simulink model "CAMFC2_Quad_New_02"  (R2017b)
settings: Solver=ode45  StartTime=0.0  StopTime=600  RelTol=1e-3  EnableMultiTasking=on
InitFcn:
  | constant_CAMFC2_Quad_New_02
values from neighbouring files (symbols this model uses):
  alpha = 0.1    [constant_CAMFC2_01_WMR01.m]    (also in constant_CAMFC2_04_Comp.m = 0.01; constant_CAMFC2_04_Quad_03.m; constant_CAMFC2_04_Simple.m = 0.01; constant_CAMFC2_04_Simple_DoubleIntegrator.m = 0.01)
  AN = [     0 1 0 0 ... (first row only)    [constant_CAMFC2_01_WMR01.m]    (also in constant_CAMFC2_04_Comp.m = [     0 1 0 0 1; constant_CAMFC2_04_Quad_03.m; constant_CAMFC2_04_Simple.m; constant_CAMFC2_04_Simple_DoubleIntegrator.m)
  B = eye(n)    [constant_CAMFC2_01_WMR01.m]    (also in constant_CAMFC2_04_Quad_03.m; constant_CAMFC2_Quad_New_02.m)
  B_pseudo_inverse = ((B'*B)^(-1))*B'    [constant_CAMFC2_01_WMR01.m]    (also in constant_CAMFC2_Quad_New_02.m)
  BBT_inv = ((B'*B)^(-1))*B'    [constant_CAMFC2_04_Quad_03.m]    (also in constant_CAMFC2_Quad_New_02.m)
  Beta = 0.2    [constant_CAMFC2_04_Quad_03.m]    (also in constant_CAMFC2_Quad_New_02.m = 0.1)
  BN = [     1 0 0 0 ... (first row only)    [constant_CAMFC2_01_WMR01.m]    (also in constant_CAMFC2_04_Comp.m = [     0 0 0 0 0; constant_CAMFC2_04_Quad_03.m; constant_CAMFC2_04_Simple.m; constant_CAMFC2_04_Simple_DoubleIntegrator.m)
  epsilon_struct = struct('data',epsilon_InitVal)    [constant_CAMFC2_01_WMR01.m]    (also in constant_CAMFC2_04_Comp.m; constant_CAMFC2_04_Quad_03.m; constant_CAMFC2_04_Simple.m; constant_CAMFC2_04_Simple_DoubleIntegrator.m)
  gama1 = 1e4*diag([1e-6*ones(2,1);1e0*ones(2,1)])    [constant_CAMFC2_01_WMR01.m]    (also in constant_CAMFC2_04_Comp.m = 1e+3*diag([1e-6;1e-0]); constant_CAMFC2_04_Quad_03.m = 1e+2*diag(1e-0*ones(n0,1)); constant_CAMFC2_04_Simple.m = 1e+2*diag([1e-0;1e-0]); constant_CAMFC2_04_Simple_Formation.m = 1e+2*diag([1e-0;1e-0]))
  gama2 = 1e-2*diag([1e-6*ones(2,1);1e0*ones(2,1)])    [constant_CAMFC2_01_WMR01.m]    (also in constant_CAMFC2_04_Comp.m = 1e+0*diag([1e-6;1e-0]); constant_CAMFC2_04_Quad_03.m = 1e+0*diag(1e-0*ones(n0,1)); constant_CAMFC2_04_Simple.m = 1e+1*diag([1e-0;1e-0]); constant_CAMFC2_04_Simple_Formation.m = 1e+1*diag([1e-0;1e-0]))
  gamma_0 = 1e+0*diag([1e-0*ones(n0,1);1e-0*ones(n0,1)])    [constant_CAMFC2_04_Quad_03.m]    (also in constant_CAMFC2_Quad_New_02.m = 1e-2*diag([1e-6*ones(n0,1);1e-0*ones(n0,1)]))
  gamma_1 = 1e+2*diag([1e-0*ones(n0,1);1e-0*ones(n0,1)])    [constant_CAMFC2_04_Quad_03.m]    (also in constant_CAMFC2_Quad_New_02.m = 1e+1*diag([1e-6*ones(n0,1);1e-0*ones(n0,1)]))
  ge = 9.81    [constant_CAMFC2_04_Comp.m]    (also in constant_CAMFC2_04_Quad_03.m; constant_CAMFC2_04_Simple.m; constant_CAMFC2_04_Simple_DoubleIntegrator.m; constant_CAMFC2_04_Simple_DoubleIntegrator_02.m)
  H = L + BN    [constant_CAMFC2_01_WMR01.m]    (also in constant_CAMFC2_04_Comp.m; constant_CAMFC2_04_Quad_03.m; constant_CAMFC2_04_Simple.m; constant_CAMFC2_04_Simple_DoubleIntegrator.m)
  J = 0.01    [constant_CAMFC2_01_WMR01.m]    (also in constant_CAMFC2_04_Quad_03.m = 1.0e-3 * diag([1 1 2],0); constant_CAMFC2_Quad_New_02.m = 1.2416e-3 * diag([1 1 2],0))
  K = 1e-2*eye(n)    [constant_CAMFC2_01_WMR01.m]    (also in constant_CAMFC2_Quad_New_02.m = 1e+1*eye(n))
  k1 = 1    [constant_CAMFC2_01_WMR01.m]    (also in constant_CAMFC2_04_Comp.m; constant_CAMFC2_04_Quad_03.m = 50; constant_CAMFC2_04_Simple.m; constant_CAMFC2_04_Simple_DoubleIntegrator.m)
  k2 = 1    [constant_CAMFC2_01_WMR01.m]    (also in constant_CAMFC2_04_Comp.m; constant_CAMFC2_04_Quad_03.m; constant_CAMFC2_04_Simple.m; constant_CAMFC2_04_Simple_DoubleIntegrator.m)
  Ka = 0.1    [constant_CAMFC2_04_Quad_03.m]    (also in constant_CAMFC2_Quad_New_02.m = 0.01)
  Kd = 0.1    [constant_CAMFC2_04_Quad_03.m]    (also in constant_CAMFC2_Quad_New_02.m = 0.01)
  Kf = 1e-5    (= 1e-05)    [constant_CAMFC2_Quad_New_02.m]
  Kt = 0.01 * Kf    (= 1e-07)    [constant_CAMFC2_Quad_New_02.m]
  Lq = 1    [constant_CAMFC2_04_Quad_03.m]    (also in constant_CAMFC2_Quad_New_02.m = 0.2)
  m = 6    [constant_CAMFC2_04_Quad_03.m]    (also in constant_CAMFC2_Quad_New_02.m)
  M = 1    [constant_CAMFC2_01_WMR01.m]    (also in constant_CAMFC2_04_Quad_03.m = 2; constant_CAMFC2_Quad_New_02.m = 2)
  N = 4    [constant_CAMFC2_01_WMR01.m]    (also in constant_CAMFC2_04_Comp.m = 5; constant_CAMFC2_04_Quad_03.m; constant_CAMFC2_04_Simple.m; constant_CAMFC2_04_Simple_DoubleIntegrator.m)
  n = 4    [constant_CAMFC2_01_WMR01.m]    (also in constant_CAMFC2_04_Comp.m = 2; constant_CAMFC2_04_Quad_03.m = 6; constant_CAMFC2_04_Simple.m = 2; constant_CAMFC2_04_Simple_DoubleIntegrator.m = 2)
  n0 = 2    [constant_CAMFC2_01_WMR01.m]    (also in constant_CAMFC2_04_Comp.m = 1; constant_CAMFC2_04_Quad_03.m = 3; constant_CAMFC2_04_Simple.m; constant_CAMFC2_04_Simple_DoubleIntegrator.m = 1)
  Observer_Gain = 100    [constant_CAMFC2_01_WMR01.m]    (also in constant_CAMFC2_04_Comp.m = 10; constant_CAMFC2_04_Quad_03.m = 1; constant_CAMFC2_04_Simple.m; constant_CAMFC2_04_Simple_DoubleIntegrator.m)
  Observer_Gain1 = 100    [constant_CAMFC2_01_WMR01.m]    (also in constant_CAMFC2_04_Comp.m = 10; constant_CAMFC2_04_Quad_03.m = 1; constant_CAMFC2_04_Simple.m; constant_CAMFC2_04_Simple_DoubleIntegrator.m)
  P_struct = struct('data',P_InitVal)    [constant_CAMFC2_01_WMR01.m]    (also in constant_CAMFC2_04_Comp.m; constant_CAMFC2_04_Quad_03.m; constant_CAMFC2_04_Simple.m; constant_CAMFC2_04_Simple_DoubleIntegrator.m)
  Q = 1e-0*eye(n)    [constant_CAMFC2_01_WMR01.m]    (also in constant_CAMFC2_04_Comp.m = 1.0e+2*eye(n); constant_CAMFC2_04_Quad_03.m = 1e-0*eye(n0); constant_CAMFC2_04_Simple.m = 1.0e+1*eye(n); constant_CAMFC2_04_Simple_Formation.m = 1.0e+1*eye(n))
  QR = 1e-0*eye(n)    [constant_CAMFC2_04_Quad_03.m]    (also in constant_CAMFC2_Quad_New_02.m = 1e+0*eye(n))
  R = 1e-0*eye(n)    [constant_CAMFC2_01_WMR01.m]    (also in constant_CAMFC2_04_Quad_03.m; constant_CAMFC2_Quad_New_02.m = 1e+0*eye(n))
  r_formX = 1.0    (= 1)    [constant_CAMFC2_04_Quad_03.m]    (also in constant_CAMFC2_Quad_New_02.m)
  r_formY = 1.0    (= 1)    [constant_CAMFC2_04_Quad_03.m]    (also in constant_CAMFC2_Quad_New_02.m)
  r_formZ = 0.5    [constant_CAMFC2_04_Quad_03.m]    (also in constant_CAMFC2_Quad_New_02.m = 1)
  rho1 = 1e-1    (= 0.1)    [constant_CAMFC2_01_WMR01.m]    (also in constant_CAMFC2_04_Comp.m = 1; constant_CAMFC2_04_Quad_03.m = 1; constant_CAMFC2_04_Simple.m = 1; constant_CAMFC2_04_Simple_DoubleIntegrator.m = 1)
  rho2 = 1e-3    (= 0.001)    [constant_CAMFC2_01_WMR01.m]    (also in constant_CAMFC2_04_Comp.m = 1; constant_CAMFC2_04_Quad_03.m = 1; constant_CAMFC2_04_Simple.m = 1; constant_CAMFC2_04_Simple_DoubleIntegrator.m = 10)
  rho_0 = 1e-0    (= 1)    [constant_CAMFC2_04_Quad_03.m]    (also in constant_CAMFC2_Quad_New_02.m = 0.01)
  rho_1 = 1e-0    (= 1)    [constant_CAMFC2_04_Quad_03.m]    (also in constant_CAMFC2_Quad_New_02.m = 0.01)
  T_struct = struct('data',T_InitVal)    [constant_CAMFC2_01_WMR01.m]    (also in constant_CAMFC2_04_Comp.m; constant_CAMFC2_04_Quad_03.m; constant_CAMFC2_04_Simple.m; constant_CAMFC2_04_Simple_DoubleIntegrator.m)
  U_dot0_M = U_dot0_m*ones(n,1)    [constant_CAMFC2_01_WMR01.m]    (also in constant_CAMFC2_Quad_New_02.m = U_dot0_m*ones(n0,1))
  Upsilon_M = Upsilon_m*ones(n,1)    [constant_CAMFC2_01_WMR01.m]    (also in constant_CAMFC2_04_Comp.m; constant_CAMFC2_04_Quad_03.m = Upsilon_m*ones(n0,1); constant_CAMFC2_04_Simple.m; constant_CAMFC2_04_Simple_DoubleIntegrator.m)
  X_M = X_m*ones(n0,1)    [constant_CAMFC2_Quad_New_02.m]
(part 3 of 3)

== matlab function CAMFC2_Quad_New_02/Agent #4/Decenteralized Cooperaive Controller #4/Cooperative Observers #1/Differentiator2/Sliding differentiator1 ==
  data: Du1 output; e input; k2 parameter; alpha parameter
function Du1 = fcn(e,k2,alpha)

a=k2;

ABS = abs(e);
SGN = e ./ (ABS + alpha);
Du1 = - a*SGN;

end

== matlab function CAMFC2_Quad_New_02/Agent #4/Decenteralized Cooperaive Controller #4/Cooperative Observers #1/Observer T#4 ==
  data: T_struct parameter; T input; DT_i output; epsilon input; epsilon_struct parameter; H parameter; BN parameter; AN parameter; T_i input; Upsilon_M parameter; epsilon_i output; N parameter; n0 parameter; Agent_Num input; Observer_Gain1 parameter; chi input
function [DT_i,epsilon_i] = fcn(T_struct,T,epsilon,epsilon_struct,H,BN,AN,T_i,Upsilon_M,N,n0,Agent_Num,Observer_Gain1, chi)

T_struct(1).data = T.t1;
T_struct(2).data = T.t2;
T_struct(3).data = T.t3;
T_struct(4).data = T.t4;

epsilon_struct(1).data = epsilon.eps1;
epsilon_struct(2).data = epsilon.eps2;
epsilon_struct(3).data = epsilon.eps3;
epsilon_struct(4).data = epsilon.eps4;

epsilon_i = + BN(Agent_Num,Agent_Num)*(T_i - chi);
Sum2 = zeros(N+1,n0);
for i=1:N
    epsilon_i = epsilon_i + ( AN(Agent_Num,i) * (T_i - T_struct(i).data) );  
    Sum2 = Sum2 + ( H(i,Agent_Num) * epsilon_struct(i).data );
end

Sum21 = abs(Sum2) + 0.1;
SGN2 = Sum2./Sum21;

DT_i = -Observer_Gain1*epsilon_i - SGN2*diag(Upsilon_M);

end

== matlab function CAMFC2_Quad_New_02/Agent #4/Decenteralized Cooperaive Controller #4/Cooperative Observers #1/Observer q#4 ==
  data: q input; Dq_i output; tau input; H parameter; BN parameter; AN parameter; q_i input; u0 input; U_dot0_M parameter; tau_i output; N parameter; Agent_Num input; Observer_Gain parameter; n0 parameter; alpha parameter
function [Dq_i,tau_i] = fcn(q,tau,H,BN,AN,q_i,u0,U_dot0_M,N,Agent_Num,Observer_Gain,n0,alpha)

tau_i = + BN(Agent_Num,Agent_Num)*(q_i - u0);
Sum2 = zeros(n0,1);
for i=1:N
    tau_i = tau_i + ( AN(Agent_Num,i) * (q_i - q(((i-1)*n0+1):n0*i)) );  
    Sum2 = Sum2 + ( H(i,Agent_Num) * tau(((i-1)*n0+1):n0*i) );
end

Sum21 = abs(Sum2) + alpha;
SGN2 = Sum2./Sum21;

Dq_i = -Observer_Gain*tau_i - diag(SGN2)*U_dot0_M;

end

== matlab function CAMFC2_Quad_New_02/Agent #4/Decenteralized Cooperaive Controller #4/Cooperative Observers #1/Observer x0_hat#4 ==
  data: x0_hat input; Dx0_hat_i output; x0_tilde input; H parameter; BN parameter; AN parameter; x0_hat_i input; x0 input; X_M parameter; x0_tilde_i output; N parameter; Agent_Num input; Observer_Gain parameter; n0 parameter; alpha parameter
function [Dx0_hat_i,x0_tilde_i] = fcn(x0_hat,x0_tilde,H,BN,AN,x0_hat_i,x0,X_M,N,Agent_Num,Observer_Gain,n0,alpha)

x0_tilde_i = + BN(Agent_Num,Agent_Num)*(x0_hat_i - x0);
Sum2 = zeros(n0,1);
for i=1:N
    x0_tilde_i = x0_tilde_i + ( AN(Agent_Num,i) * (x0_hat_i - x0_hat(((i-1)*n0+1):n0*i)) );  
    Sum2 = Sum2 + ( H(i,Agent_Num) * x0_tilde(((i-1)*n0+1):n0*i) );
end

Sum21 = abs(Sum2) + alpha;
SGN2 = Sum2./Sum21;

Dx0_hat_i = -Observer_Gain*x0_tilde_i - diag(SGN2)*X_M;

end

== matlab function CAMFC2_Quad_New_02/Agent #4/Decenteralized Cooperaive Controller #4/Rotational/Differentiator/Sliding differentiator1 ==
  data: Du1 output; e input; n parameter; k2 parameter
function Du1 = fcn(e,n,k2)

a=k2;

ABS = zeros(n,1);
for i=1:n
    if e(i)>0
        ABS(i) = e(i);
    else
        ABS(i) = -e(i);
    end
end
SGN = e ./ (ABS + 0.01);

Du1 = - a*SGN;

end

== matlab function CAMFC2_Quad_New_02/Agent #4/Decenteralized Cooperaive Controller #4/Rotational/g-Estimator ==
  data: sigma input; g_hat input; P input; rho_1 parameter; gamma_1 parameter; Dg_hat output
function Dg_hat = fcn(sigma,g_hat,P,rho_1,gamma_1)

Dg_hat = - gamma_1 * P * sigma - rho_1 * gamma_1 * g_hat;

end

== matlab function CAMFC2_Quad_New_02/Agent #4/Decenteralized Cooperaive Controller #4/Rotational/g-Estimator1 ==
  data: sigma input; x input; P input; rho_0 parameter; gamma_0 parameter; Da_hat output; a_hat input
function Da_hat = fcn(sigma,x,P,rho_0,gamma_0,a_hat)

DVa_hat = - gamma_0 * P * diag(sigma) * (x - sigma) - rho_0 * gamma_0 * diag(a_hat);

Da_hat = diag(DVa_hat);

end

== matlab function CAMFC2_Quad_New_02/Agent #4/Decenteralized Cooperaive Controller #4/Rotational/main ==
  data: sigma input; zeta input; u output; Dy_d input; R parameter; P input; a_hat input; B parameter; g_hat input; x input; QR parameter; BBT_inv parameter; n parameter
function u = fcn(sigma,zeta,Dy_d,R,P,a_hat,B,g_hat,x,QR,BBT_inv,n)

u1 = (1/2) * R * B' * P * sigma;
u2 = BBT_inv * (Dy_d - a_hat*x + (eye(n) + 2*(((P)^(-1)*QR)) + a_hat)*sigma - g_hat - zeta) - (3/4) * R * B' * P * sigma;

u = u1 + u2;

end

== matlab function CAMFC2_Quad_New_02/Agent #4/Decenteralized Cooperaive Controller #4/Rotational/variable change ==
  data: X input; Xd input; x_mod output; u input; xd_mod output; e_mod output
function [x_mod,xd_mod,e_mod] = fcn(X,Xd,u)

x_mod = [X(4:6);X(10:12)];

xd_mod = [Xd;u(1:3)];

e_mod = xd_mod - x_mod;


end

== matlab function CAMFC2_Quad_New_02/Agent #1/Decenteralized Cooperaive Controller #1/Rotational/CARE ==
  data: P input; a_hat input; B parameter; R parameter; DP output; QR parameter
function DP = fcn(P,a_hat,B,R,QR)

DP = a_hat*P + P*a_hat' - P*B*R*B'*P + 2*QR;

end

== matlab function CAMFC2_Quad_New_02/Data Bus /Reference Trajectory/Differentiator0/Sliding differentiator ==
  data: u output; u1 input; e input; k1 parameter; alpha parameter
function u = fcn(u1,e,k1,alpha)

b=k1;

ABS = abs(e);
SGN = e ./ (ABS + alpha);
u = u1 - b*((ABS.^0.5).*SGN); 

end

== matlab function CAMFC2_Quad_New_02/Data Bus /Translational Log/For matrix Plot1/MATLAB Function ==
  data: u input; y output
function y = fcn(u)
S1 = size(u,1);
S2 = size(u,2);

y = zeros(S1*S2,1);
num = 0;
for i=1:S1
    for j=1:S2
        num = num + 1;
        y(num,1) = u(i,j);
    end
end

end

== matlab function CAMFC2_Quad_New_02/Data Bus /Translational Log/For matrix Plot2/MATLAB Function ==
  data: u input; y output
function y = fcn(u)
S1 = size(u,1);
S2 = size(u,2);

y = zeros(S1*S2,1);
num = 0;
for i=1:S1
    for j=1:S2
        num = num + 1;
        y(num,1) = u(i,j);
    end
end

end

== matlab function CAMFC2_Quad_New_02/Data Bus /Translational Log/For matrix Plot3/MATLAB Function ==
  data: u input; y output
function y = fcn(u)
S1 = size(u,1);
S2 = size(u,2);

y = zeros(S1*S2,1);
num = 0;
for i=1:S1
    for j=1:S2
        num = num + 1;
        y(num,1) = u(i,j);
    end
end

end

== matlab function CAMFC2_Quad_New_02/Data Bus /Translational Log/For matrix Plot4/MATLAB Function ==
  data: u input; y output
function y = fcn(u)
S1 = size(u,1);
S2 = size(u,2);

y = zeros(S1*S2,1);
num = 0;
for i=1:S1
    for j=1:S2
        num = num + 1;
        y(num,1) = u(i,j);
    end
end

end

== matlab function CAMFC2_Quad_New_02/Data Bus /Translational Log/For matrix Plot5/MATLAB Function ==
  data: u input; y output
function y = fcn(u)
S1 = size(u,1);
S2 = size(u,2);

y = zeros(S1*S2,1);
num = 0;
for i=1:S1
    for j=1:S2
        num = num + 1;
        y(num,1) = u(i,j);
    end
end

end

== matlab function CAMFC2_Quad_New_02/Data Bus /Translational Log/For matrix Plot6/MATLAB Function ==
  data: u input; y output
function y = fcn(u)
S1 = size(u,1);
S2 = size(u,2);

y = zeros(S1*S2,1);
num = 0;
for i=1:S1
    for j=1:S2
        num = num + 1;
        y(num,1) = u(i,j);
    end
end

end

== matlab function CAMFC2_Quad_New_02/Data Bus /Translational Log/For matrix Plot7/MATLAB Function ==
  data: u input; y output
function y = fcn(u)
S1 = size(u,1);
S2 = size(u,2);

y = zeros(S1*S2,1);
num = 0;
for i=1:S1
    for j=1:S2
        num = num + 1;
        y(num,1) = u(i,j);
    end
end

end

== matlab function CAMFC2_Quad_New_02/Data Bus /Observers Log/For matrix Plot8/MATLAB Function ==
  data: u input; y output
function y = fcn(u)
S1 = size(u,1);
S2 = size(u,2);

y = zeros(S1*S2,1);
num = 0;
for i=1:S1
    for j=1:S2
        num = num + 1;
        y(num,1) = u(i,j);
    end
end

end

== matlab function CAMFC2_Quad_New_02/Data Bus /Observers Log/For matrix Plot9/MATLAB Function ==
  data: u input; y output
function y = fcn(u)
S1 = size(u,1);
S2 = size(u,2);

y = zeros(S1*S2,1);
num = 0;
for i=1:S1
    for j=1:S2
        num = num + 1;
        y(num,1) = u(i,j);
    end
end

end

== matlab function CAMFC2_Quad_New_02/Agent #2/Decenteralized Cooperaive Controller #2/Rotational/CARE ==
  data: P input; a_hat input; B parameter; R parameter; DP output; QR parameter
function DP = fcn(P,a_hat,B,R,QR)

DP = a_hat*P + P*a_hat' - P*B*R*B'*P + 2*QR;

end

== matlab function CAMFC2_Quad_New_02/Agent #2/Decenteralized Cooperaive Controller #2/Rotational/Differentiator/Sliding differentiator ==
  data: u output; u1 input; e input; n parameter; k1 parameter
function u = fcn(u1,e,n,k1)

b=k1;

ABS = zeros(n,1);
for i=1:n
    if e(i)>0
        ABS(i) = e(i);
    else
        ABS(i) = -e(i);
    end
end
SGN = e ./ (ABS + 0.01);

u = u1 - b*(ABS.^0.5).*SGN;

end

== matlab function CAMFC2_Quad_New_02/Data Bus /Translational Log/For matrix Plot/MATLAB Function ==
  data: u input; y output
function y = fcn(u)
S1 = size(u,1);
S2 = size(u,2);

y = zeros(S1*S2,1);
num = 0;
for i=1:S1
    for j=1:S2
        num = num + 1;
        y(num,1) = u(i,j);
    end
end

end

== matlab function CAMFC2_Quad_New_02/Data Bus /Observers Log/For matrix Plot10/MATLAB Function ==
  data: u input; y output
function y = fcn(u)
S1 = size(u,1);
S2 = size(u,2);

y = zeros(S1*S2,1);
num = 0;
for i=1:S1
    for j=1:S2
        num = num + 1;
        y(num,1) = u(i,j);
    end
end

end

== matlab function CAMFC2_Quad_New_02/Data Bus /Observers Log/For matrix Plot11/MATLAB Function ==
  data: u input; y output
function y = fcn(u)
S1 = size(u,1);
S2 = size(u,2);

y = zeros(S1*S2,1);
num = 0;
for i=1:S1
    for j=1:S2
        num = num + 1;
        y(num,1) = u(i,j);
    end
end

end

== matlab function CAMFC2_Quad_New_02/Data Bus /Observers Log/For matrix Plot12/MATLAB Function ==
  data: u input; y output
function y = fcn(u)
S1 = size(u,1);
S2 = size(u,2);

y = zeros(S1*S2,1);
num = 0;
for i=1:S1
    for j=1:S2
        num = num + 1;
        y(num,1) = u(i,j);
    end
end

end

== matlab function CAMFC2_Quad_New_02/Agent #2/Decenteralized Cooperaive Controller #2/Rotational/Differentiator/Sliding differentiator1 ==
  data: Du1 output; e input; n parameter; k2 parameter
function Du1 = fcn(e,n,k2)

a=k2;

ABS = zeros(n,1);
for i=1:n
    if e(i)>0
        ABS(i) = e(i);
    else
        ABS(i) = -e(i);
    end
end
SGN = e ./ (ABS + 0.01);

Du1 = - a*SGN;

end

== matlab function CAMFC2_Quad_New_02/Data Bus /Observers Log/For matrix Plot13/MATLAB Function ==
  data: u input; y output
function y = fcn(u)
S1 = size(u,1);
S2 = size(u,2);

y = zeros(S1*S2,1);
num = 0;
for i=1:S1
    for j=1:S2
        num = num + 1;
        y(num,1) = u(i,j);
    end
end

end

== matlab function CAMFC2_Quad_New_02/Agent #2/Decenteralized Cooperaive Controller #2/Rotational/g-Estimator ==
  data: sigma input; g_hat input; P input; rho_1 parameter; gamma_1 parameter; Dg_hat output
function Dg_hat = fcn(sigma,g_hat,P,rho_1,gamma_1)

Dg_hat = - gamma_1 * P * sigma - rho_1 * gamma_1 * g_hat;

end

== matlab function CAMFC2_Quad_New_02/Agent #4/Plant #4/MATLAB Function ==
  data: X input; U input; t input; DX output; Kf parameter; Kt parameter; Kd parameter; Ka parameter; M parameter; J parameter; Lq parameter; ge parameter
function DX = fcn(X,U,t,Kf,Kt,Kd,Ka,M,J,Lq,ge)

phi = X(4);
theta = X(5);
psi = X(6);

Rq = [cos(psi)*cos(theta) -sin(psi)*cos(phi)+cos(psi)*sin(theta)*sin(phi) sin(psi)*sin(phi)+cos(psi)*sin(theta)*cos(phi);
    sin(psi)*cos(theta) cos(psi)*cos(phi)+sin(psi)*sin(theta)*sin(phi) -cos(psi)*sin(phi)+sin(psi)*sin(theta)*cos(phi);
    -sin(theta) cos(theta)*sin(phi) cos(theta)*cos(phi)]; 

R_omega = [1 0 -sin(theta);
    0 cos(phi) cos(theta)*sin(phi);
    0 -sin(phi) cos(theta)*cos(phi)];

EXT_PRD = External_Product3(X(10:12),(J*X(10:12)));

F1 = Kf * U(1)^2;
F2 = Kf * U(2)^2;
F3 = Kf * U(3)^2;
F4 = Kf * U(4)^2;
  
FT = F1 + F2 + F3 + F4;
 
T1 = Kt * U(1)^2;
T2 = Kt * U(2)^2;
T3 = Kt * U(3)^2;
T4 = Kt * U(4)^2;
 
TT1 = Lq*(F3-F1);
TT2 = Lq*(F4-F2);
TT3 = (T1-T2+T3-T4);

FTT = Rq * [0;0;FT];
FTx = FTT(1);
FTy = FTT(2);
FTz = FTT(3);

DP = X(7:9);
DPHI = (R_omega)^(-1) * X(10:12); 
Dv = (1/M)*([FTx;FTy;FTz] - Kd*X(7:9) - M*[0;0;ge]) + Rq*(0.1*sin(1*t))*[0;0;1]; 
Dw = (J^(-1))*([TT1;TT2;TT3] - Ka*X(10:12) - EXT_PRD) + (1*sin(1*t)*[1;1;1]);

DX = [DP;DPHI;Dv;Dw];

end

== matlab function CAMFC2_Quad_New_02/Data Bus /Observers Log/For matrix Plot14/MATLAB Function ==
  data: u input; y output
function y = fcn(u)
S1 = size(u,1);
S2 = size(u,2);

y = zeros(S1*S2,1);
num = 0;
for i=1:S1
    for j=1:S2
        num = num + 1;
        y(num,1) = u(i,j);
    end
end

end

== matlab function CAMFC2_Quad_New_02/Data Bus /Observers Log/For matrix Plot15/MATLAB Function ==
  data: u input; y output
function y = fcn(u)
S1 = size(u,1);
S2 = size(u,2);

y = zeros(S1*S2,1);
num = 0;
for i=1:S1
    for j=1:S2
        num = num + 1;
        y(num,1) = u(i,j);
    end
end

end

== matlab function CAMFC2_Quad_New_02/Data Bus /Reference Trajectory/Differentiator0/Sliding differentiator1 ==
  data: Du1 output; e input; k2 parameter; alpha parameter
function Du1 = fcn(e,k2,alpha)

a=k2;

ABS = abs(e);
SGN = e ./ (ABS + alpha);
Du1 = - a*SGN;

end

== matlab function CAMFC2_Quad_New_02/Data Bus /Reference Trajectory/MATLAB Function ==
  data: r_formZ_inp input; chi output; r_formX_inp input; r_formY_inp input
function chi = fcn(r_formZ_inp, r_formX_inp, r_formY_inp)

Delta_form = [...
    +r_formX_inp +r_formY_inp +r_formZ_inp;
    -r_formX_inp +r_formY_inp +2*r_formZ_inp;
    -r_formX_inp -r_formY_inp +3*r_formZ_inp;
    +r_formX_inp -r_formY_inp +4*r_formZ_inp];

chi = [0 0 0;
    Delta_form];

end

== matlab function CAMFC2_Quad_New_02/Agent #1/Decenteralized Cooperaive Controller #1/Rotational/Differentiator/Sliding differentiator ==
  data: u output; u1 input; e input; n parameter; k1 parameter
function u = fcn(u1,e,n,k1)

b=k1;

ABS = zeros(n,1);
for i=1:n
    if e(i)>0
        ABS(i) = e(i);
    else
        ABS(i) = -e(i);
    end
end
SGN = e ./ (ABS + 0.01);

u = u1 - b*(ABS.^0.5).*SGN;

end

== matlab function CAMFC2_Quad_New_02/Agent #4/Decenteralized Cooperaive Controller #4/Translational #4/Adaptive Law A_T #4 ==
  data: Agent_Num input; A_hat input; gama2 parameter; rho2 parameter; T_i input; P_i input; DA_hat output; e_i input; H parameter; BN parameter; N parameter; n parameter; n0 parameter; z0 input; x0_hat_inp input; ui input
function DA_hat = fcn(Agent_Num,A_hat,gama2,rho2,T_i,P_i,e_i,H,BN,N,n,n0,z0,x0_hat_inp,ui)

%% 
z0_i = [z0;ui(1:n0)]; 
x0_hat_i = [x0_hat_inp;ui(1:n0)];

%%
vA_hat = diag(A_hat);

Sum = zeros(n,1);
for i=2:(N+1)
    Sum = Sum + ( H(Agent_Num,(i-1)) * ( (2*x0_hat_i) - (2*[T_i(1,:)';zeros(n0,1)]) + ([T_i(i,:)';zeros(n0,1)]) ) );
end
Sum(1:n0) = Sum(1:n0) + ( BN(Agent_Num,Agent_Num)*z0_i(1:n0) ) - e_i(1:n0);
Sum(n0+1:n) = Sum(n0+1:n) + ( 1*z0_i(n0+1:n) ) - e_i(n0+1:n);
    
DvA_hat = -gama2*diag(Sum)*P_i * e_i - (rho2*gama2*vA_hat);

DA_hat = diag(DvA_hat);

end

== matlab function CAMFC2_Quad_New_02/Agent #4/Decenteralized Cooperaive Controller #4/Translational #4/Adaptive Law g_T #4 ==
  data: Agent_Num input; g_hat input; gama1 parameter; rho1 parameter; P input; P_struct parameter; Dg_hat output; e input; H parameter; N parameter; n parameter
function Dg_hat = fcn(Agent_Num,g_hat,gama1,rho1,P,P_struct,e,H,N,n)

P_struct(1).data = P.p1;
P_struct(2).data = P.p2;
P_struct(3).data = P.p3;
P_struct(4).data = P.p4;

Sum = zeros(n,1);
for i=1:N  
    Sum = Sum + (H(i,Agent_Num) * P_struct(i).data * e((i-1)*n+1:(i*n),1)); %Adaptive law
end
    
Dg_hat = -gama1*Sum - (rho1*gama1*g_hat);

end

== matlab function CAMFC2_Quad_New_02/Agent #4/Decenteralized Cooperaive Controller #4/Translational #4/DRE_T ==
  data: P input; A_hat input; B parameter; R parameter; DP output; Q parameter
function DP = fcn(P,A_hat,B,R,Q)

DP = 2*A_hat*P + 2*P*A_hat' - P*B*R*B'*P + 2*Q;

end

== matlab function CAMFC2_Quad_New_02/Agent #4/Decenteralized Cooperaive Controller #4/Translational #4/Differentiator1/Sliding differentiator ==
  data: u output; u1 input; e input; k1 parameter; alpha parameter
function u = fcn(u1,e,k1,alpha)

b=k1;

ABS = abs(e);
SGN = e ./ (ABS + alpha);
u = u1 - b*((ABS.^0.5).*SGN); 

end

== matlab function CAMFC2_Quad_New_02/Agent #4/Decenteralized Cooperaive Controller #4/Translational #4/Differentiator1/Sliding differentiator1 ==
  data: Du1 output; e input; k2 parameter; alpha parameter
function Du1 = fcn(e,k2,alpha)

a=k2;

ABS = abs(e);
SGN = e ./ (ABS + alpha);
Du1 = - a*SGN;

end

== matlab function CAMFC2_Quad_New_02/Agent #4/Decenteralized Cooperaive Controller #4/Translational #4/Main Controller_T #4 ==
  data: n parameter; n0 parameter; U output; R parameter; Q parameter; P_i input; e_i input; K parameter; Zeta_i input; BN parameter; A_hat_i input; u0 input; z0 input; DT_i input; T_i input; H parameter; q_i input; Agent_Num input; B_pseudo_inverse parameter; ui input; x0_hat_inp input; g_hat_i input; D_ui1 input
function U = fcn(n,n0,R,Q,P_i,e_i,K,Zeta_i,BN,A_hat_i,u0,z0,DT_i,T_i,H,q_i,Agent_Num,B_pseudo_inverse,ui,x0_hat_inp, g_hat_i, D_ui1)

D_eta_0 = [DT_i(1,:)';zeros(n0,1)];

%% 
z0_i = [z0;ui(1:n0)];
x0_hat_i = [x0_hat_inp;ui(1:n0)];
u0_i = [u0;D_ui1];

%%

S_H = sum(H(Agent_Num,:)) - H(Agent_Num,Agent_Num);
U4 = - S_H * ([q_i;u0_i(n0+1:n)] - [DT_i(1,:)';zeros(n0,1)] - (A_hat_i * (x0_hat_i - [T_i(1,:)';zeros(n0,1)])));
U1 = 1/2 * R * P_i * e_i; %Consensus Error
U5 = ( A_hat_i * ( H(Agent_Num,Agent_Num)*(2*x0_hat_i - 2*[T_i(1,:)';zeros(n0,1)] + [T_i(Agent_Num+1,:)';zeros(n0,1)]) ) ) - e_i;
U5(1:n0) = U5(1:n0) + ( BN(Agent_Num,Agent_Num) * z0_i(1:n0) );
U5(n0+1:n) = U5(n0+1:n) + ( 1 * z0_i(n0+1:n) );
U2 = - g_hat_i; %nonlinear compensation 
U3 = + [DT_i(Agent_Num+1,:)';zeros(n0,1)]; %Derivative of Formation parameters  
U6 = zeros(n,1);
U6(1:n0) = - BN(Agent_Num,Agent_Num)*( D_eta_0(1:n0) - u0_i(1:n0) ); %Connection to the leader
U6(n0+1:n) = - 1 * ( D_eta_0(n0+1:n) - u0_i(n0+1:n) );
U7 = K * Zeta_i; %Consensus time-integral
U8 = (2*Q - 3/4*R*P_i)*e_i;

U_input = U1 + U2 + U3 + U4 + U5 + U6 + U7 + U8;

U = B_pseudo_inverse * U_input / H(Agent_Num,Agent_Num);

end

== matlab function CAMFC2_Quad_New_02/Agent #1/Decenteralized Cooperaive Controller #1/Controller Interpreter #1 ==
  data: ut_i input; uT_i output; PHI_d_i output
function [uT_i,PHI_d_i] = fcn(ut_i)

%%
f0 = sqrt((ut_i(4)^2)+(ut_i(5)^2)+(ut_i(6)^2));
psi_d = 0;
phi_d = asin( min(max(((sin(psi_d)*ut_i(4) - cos(psi_d)*ut_i(5)) / (f0+1e-3)),-1),1) );
theta_d = atan( (cos(psi_d)*ut_i(4) + sin(psi_d)*ut_i(5)) / (ut_i(6)+1e-3) );
PHI_d_i = [phi_d;theta_d;psi_d]; 
uT_i = f0;

end

== matlab function CAMFC2_Quad_New_02/Agent #1/Decenteralized Cooperaive Controller #1/Rotational/Differentiator/Sliding differentiator1 ==
  data: Du1 output; e input; n parameter; k2 parameter
function Du1 = fcn(e,n,k2)

a=k2;

ABS = zeros(n,1);
for i=1:n
    if e(i)>0
        ABS(i) = e(i);
    else
        ABS(i) = -e(i);
    end
end
SGN = e ./ (ABS + 0.01);

Du1 = - a*SGN;

end

== matlab function CAMFC2_Quad_New_02/Agent #1/Decenteralized Cooperaive Controller #1/Rotational/g-Estimator ==
  data: sigma input; g_hat input; P input; rho_1 parameter; gamma_1 parameter; Dg_hat output
function Dg_hat = fcn(sigma,g_hat,P,rho_1,gamma_1)

Dg_hat = - gamma_1 * P * sigma - rho_1 * gamma_1 * g_hat;

end

== matlab function CAMFC2_Quad_New_02/Agent #1/Decenteralized Cooperaive Controller #1/Rotational/g-Estimator1 ==
  data: sigma input; x input; P input; rho_0 parameter; gamma_0 parameter; Da_hat output; a_hat input
function Da_hat = fcn(sigma,x,P,rho_0,gamma_0,a_hat)

DVa_hat = - gamma_0 * P * diag(sigma) * (x - sigma) - rho_0 * gamma_0 * diag(a_hat);

Da_hat = diag(DVa_hat);

end

== matlab function CAMFC2_Quad_New_02/Agent #1/Decenteralized Cooperaive Controller #1/Rotational/main ==
  data: sigma input; zeta input; u output; Dy_d input; R parameter; P input; a_hat input; B parameter; g_hat input; x input; QR parameter; BBT_inv parameter; n parameter
function u = fcn(sigma,zeta,Dy_d,R,P,a_hat,B,g_hat,x,QR,BBT_inv,n)

u1 = (1/2) * R * B' * P * sigma;
u2 = BBT_inv * (Dy_d - a_hat*x + (eye(n) + 2*(((P)^(-1)*QR)) + a_hat)*sigma - g_hat - zeta) - (3/4) * R * B' * P * sigma;

u = u1 + u2;

end

== matlab function CAMFC2_Quad_New_02/Agent #1/Decenteralized Cooperaive Controller #1/Rotational/variable change ==
  data: X input; Xd input; x_mod output; u input; xd_mod output; e_mod output
function [x_mod,xd_mod,e_mod] = fcn(X,Xd,u)

x_mod = [X(4:6);X(10:12)];

xd_mod = [Xd;u(1:3)];

e_mod = xd_mod - x_mod;


end

== matlab function CAMFC2_Quad_New_02/Agent #2/Decenteralized Cooperaive Controller #2/Rotational/g-Estimator1 ==
  data: sigma input; x input; P input; rho_0 parameter; gamma_0 parameter; Da_hat output; a_hat input
function Da_hat = fcn(sigma,x,P,rho_0,gamma_0,a_hat)

DVa_hat = - gamma_0 * P * diag(sigma) * (x - sigma) - rho_0 * gamma_0 * diag(a_hat);

Da_hat = diag(DVa_hat);

end

== matlab function CAMFC2_Quad_New_02/Agent #2/Decenteralized Cooperaive Controller #2/Rotational/main ==
  data: sigma input; zeta input; u output; Dy_d input; R parameter; P input; a_hat input; B parameter; g_hat input; x input; QR parameter; BBT_inv parameter; n parameter
function u = fcn(sigma,zeta,Dy_d,R,P,a_hat,B,g_hat,x,QR,BBT_inv,n)

u1 = (1/2) * R * B' * P * sigma;
u2 = BBT_inv * (Dy_d - a_hat*x + (eye(n) + 2*(((P)^(-1)*QR)) + a_hat)*sigma - g_hat - zeta) - (3/4) * R * B' * P * sigma;

u = u1 + u2;

end

== matlab function CAMFC2_Quad_New_02/Agent #2/Decenteralized Cooperaive Controller #2/Rotational/variable change ==
  data: X input; Xd input; x_mod output; u input; xd_mod output; e_mod output
function [x_mod,xd_mod,e_mod] = fcn(X,Xd,u)

x_mod = [X(4:6);X(10:12)];

xd_mod = [Xd;u(1:3)];

e_mod = xd_mod - x_mod;


end

== matlab function CAMFC2_Quad_New_02/Agent #2/Decenteralized Cooperaive Controller #2/Cooperative Observers #2/Observer q#2 ==
  data: q input; Dq_i output; tau input; H parameter; BN parameter; AN parameter; q_i input; u0 input; U_dot0_M parameter; tau_i output; N parameter; Agent_Num input; Observer_Gain parameter; n0 parameter; alpha parameter
function [Dq_i,tau_i] = fcn(q,tau,H,BN,AN,q_i,u0,U_dot0_M,N,Agent_Num,Observer_Gain,n0,alpha)

tau_i = + BN(Agent_Num,Agent_Num)*(q_i - u0);
Sum2 = zeros(n0,1);
for i=1:N
    tau_i = tau_i + ( AN(Agent_Num,i) * (q_i - q(((i-1)*n0+1):n0*i)) );  
    Sum2 = Sum2 + ( H(i,Agent_Num) * tau(((i-1)*n0+1):n0*i) );
end

Sum21 = abs(Sum2) + alpha;
SGN2 = Sum2./Sum21;

Dq_i = -Observer_Gain*tau_i - diag(SGN2)*U_dot0_M;

end

== matlab function CAMFC2_Quad_New_02/Data Bus /Rotational Log/For matrix Plot/MATLAB Function ==
  data: u input; y output
function y = fcn(u)
S1 = size(u,1);
S2 = size(u,2);

y = zeros(S1*S2,1);
num = 0;
for i=1:S1
    for j=1:S2
        num = num + 1;
        y(num,1) = u(i,j);
    end
end

end

== matlab function CAMFC2_Quad_New_02/Data Bus /Rotational Log/For matrix Plot1/MATLAB Function ==
  data: u input; y output
function y = fcn(u)
S1 = size(u,1);
S2 = size(u,2);

y = zeros(S1*S2,1);
num = 0;
for i=1:S1
    for j=1:S2
        num = num + 1;
        y(num,1) = u(i,j);
    end
end

end

== matlab function CAMFC2_Quad_New_02/Data Bus /Rotational Log/For matrix Plot2/MATLAB Function ==
  data: u input; y output
function y = fcn(u)
S1 = size(u,1);
S2 = size(u,2);

y = zeros(S1*S2,1);
num = 0;
for i=1:S1
    for j=1:S2
        num = num + 1;
        y(num,1) = u(i,j);
    end
end

end

== matlab function CAMFC2_Quad_New_02/Data Bus /Rotational Log/For matrix Plot3/MATLAB Function ==
  data: u input; y output
function y = fcn(u)
S1 = size(u,1);
S2 = size(u,2);

y = zeros(S1*S2,1);
num = 0;
for i=1:S1
    for j=1:S2
        num = num + 1;
        y(num,1) = u(i,j);
    end
end

end

== matlab function CAMFC2_Quad_New_02/Data Bus /Rotational Log/For matrix Plot4/MATLAB Function ==
  data: u input; y output
function y = fcn(u)
S1 = size(u,1);
S2 = size(u,2);

y = zeros(S1*S2,1);
num = 0;
for i=1:S1
    for j=1:S2
        num = num + 1;
        y(num,1) = u(i,j);
    end
end

end

== matlab function CAMFC2_Quad_New_02/Data Bus /Rotational Log/For matrix Plot5/MATLAB Function ==
  data: u input; y output
function y = fcn(u)
S1 = size(u,1);
S2 = size(u,2);

y = zeros(S1*S2,1);
num = 0;
for i=1:S1
    for j=1:S2
        num = num + 1;
        y(num,1) = u(i,j);
    end
end

end

== matlab function CAMFC2_Quad_New_02/Agent #2/Decenteralized Cooperaive Controller #2/Controller Interpreter #2 ==
  data: ut_i input; uT_i output; PHI_d_i output
function [uT_i,PHI_d_i] = fcn(ut_i)

%%
f0 = sqrt((ut_i(4)^2)+(ut_i(5)^2)+(ut_i(6)^2));
psi_d = 0;
phi_d = asin( min(max(((sin(psi_d)*ut_i(4) - cos(psi_d)*ut_i(5)) / (f0+1e-3)),-1),1) );
theta_d = atan( (cos(psi_d)*ut_i(4) + sin(psi_d)*ut_i(5)) / (ut_i(6)+1e-3) );
PHI_d_i = [phi_d;theta_d;psi_d]; 
uT_i = f0;

end

== matlab function CAMFC2_Quad_New_02/Agent #2/Decenteralized Cooperaive Controller #2/Controller To Motors #2 ==
  data: u output; uT input; uR input; RM_1 parameter
function u = fcn(uT,uR,RM_1)

y1 = uR(4);
y2 = uR(5);
y3 = uR(6);

Y = [uT;y1;y2;y3];

u = RM_1*Y;

for i=1:4
    u(i) = sqrt(abs(u(i)));
end

end

== matlab function CAMFC2_Quad_New_02/Agent #2/Decenteralized Cooperaive Controller #2/Cooperative Observers #2/Differentiator2/Sliding differentiator ==
  data: u output; u1 input; e input; k1 parameter; alpha parameter
function u = fcn(u1,e,k1,alpha)

b=k1;

ABS = abs(e);
SGN = e ./ (ABS + alpha);
u = u1 - b*((ABS.^0.5).*SGN); 

end

== matlab function CAMFC2_Quad_New_02/Agent #2/Decenteralized Cooperaive Controller #2/Cooperative Observers #2/Differentiator2/Sliding differentiator1 ==
  data: Du1 output; e input; k2 parameter; alpha parameter
function Du1 = fcn(e,k2,alpha)

a=k2;

ABS = abs(e);
SGN = e ./ (ABS + alpha);
Du1 = - a*SGN;

end

== matlab function CAMFC2_Quad_New_02/Agent #2/Decenteralized Cooperaive Controller #2/Cooperative Observers #2/Observer T#2 ==
  data: T_struct parameter; T input; DT_i output; epsilon input; epsilon_struct parameter; H parameter; BN parameter; AN parameter; T_i input; Upsilon_M parameter; epsilon_i output; N parameter; n0 parameter; Agent_Num input; Observer_Gain1 parameter; chi input
function [DT_i,epsilon_i] = fcn(T_struct,T,epsilon,epsilon_struct,H,BN,AN,T_i,Upsilon_M,N,n0,Agent_Num,Observer_Gain1, chi)

T_struct(1).data = T.t1;
T_struct(2).data = T.t2;
T_struct(3).data = T.t3;
T_struct(4).data = T.t4;

epsilon_struct(1).data = epsilon.eps1;
epsilon_struct(2).data = epsilon.eps2;
epsilon_struct(3).data = epsilon.eps3;
epsilon_struct(4).data = epsilon.eps4;

epsilon_i = + BN(Agent_Num,Agent_Num)*(T_i - chi);
Sum2 = zeros(N+1,n0);
for i=1:N
    epsilon_i = epsilon_i + ( AN(Agent_Num,i) * (T_i - T_struct(i).data) );  
    Sum2 = Sum2 + ( H(i,Agent_Num) * epsilon_struct(i).data );
end

Sum21 = abs(Sum2) + 0.1;
SGN2 = Sum2./Sum21;

DT_i = -Observer_Gain1*epsilon_i - SGN2*diag(Upsilon_M);

end

== matlab function CAMFC2_Quad_New_02/Data Bus /Rotational Log/For matrix Plot6/MATLAB Function ==
  data: u input; y output
function y = fcn(u)
S1 = size(u,1);
S2 = size(u,2);

y = zeros(S1*S2,1);
num = 0;
for i=1:S1
    for j=1:S2
        num = num + 1;
        y(num,1) = u(i,j);
    end
end

end

== matlab function CAMFC2_Quad_New_02/Agent #2/Decenteralized Cooperaive Controller #2/Cooperative Observers #2/Observer x0_hat#2 ==
  data: x0_hat input; Dx0_hat_i output; x0_tilde input; H parameter; BN parameter; AN parameter; x0_hat_i input; x0 input; X_M parameter; x0_tilde_i output; N parameter; Agent_Num input; Observer_Gain parameter; n0 parameter; alpha parameter
function [Dx0_hat_i,x0_tilde_i] = fcn(x0_hat,x0_tilde,H,BN,AN,x0_hat_i,x0,X_M,N,Agent_Num,Observer_Gain,n0,alpha)

x0_tilde_i = + BN(Agent_Num,Agent_Num)*(x0_hat_i - x0);
Sum2 = zeros(n0,1);
for i=1:N
    x0_tilde_i = x0_tilde_i + ( AN(Agent_Num,i) * (x0_hat_i - x0_hat(((i-1)*n0+1):n0*i)) );  
    Sum2 = Sum2 + ( H(i,Agent_Num) * x0_tilde(((i-1)*n0+1):n0*i) );
end

Sum21 = abs(Sum2) + alpha;
SGN2 = Sum2./Sum21;

Dx0_hat_i = -Observer_Gain*x0_tilde_i - diag(SGN2)*X_M;

end

== matlab function CAMFC2_Quad_New_02/Data Bus /Rotational Log/For matrix Plot7/MATLAB Function ==
  data: u input; y output
function y = fcn(u)
S1 = size(u,1);
S2 = size(u,2);

y = zeros(S1*S2,1);
num = 0;
for i=1:S1
    for j=1:S2
        num = num + 1;
        y(num,1) = u(i,j);
    end
end

end

== matlab function CAMFC2_Quad_New_02/Agent #2/Decenteralized Cooperaive Controller #2/Translational #2/Adaptive Law A_T #2 ==
  data: Agent_Num input; A_hat input; gama2 parameter; rho2 parameter; T_i input; P_i input; DA_hat output; e_i input; H parameter; BN parameter; N parameter; n parameter; n0 parameter; z0 input; x0_hat_inp input; ui input
function DA_hat = fcn(Agent_Num,A_hat,gama2,rho2,T_i,P_i,e_i,H,BN,N,n,n0,z0,x0_hat_inp,ui)

%% 
z0_i = [z0;ui(1:n0)]; 
x0_hat_i = [x0_hat_inp;ui(1:n0)];

%%
vA_hat = diag(A_hat);

Sum = zeros(n,1);
for i=2:(N+1)
    Sum = Sum + ( H(Agent_Num,(i-1)) * ( (2*x0_hat_i) - (2*[T_i(1,:)';zeros(n0,1)]) + ([T_i(i,:)';zeros(n0,1)]) ) );
end
Sum(1:n0) = Sum(1:n0) + ( BN(Agent_Num,Agent_Num)*z0_i(1:n0) ) - e_i(1:n0);
Sum(n0+1:n) = Sum(n0+1:n) + ( 1*z0_i(n0+1:n) ) - e_i(n0+1:n);
    
DvA_hat = -gama2*diag(Sum)*P_i * e_i - (rho2*gama2*vA_hat);

DA_hat = diag(DvA_hat);

end

== matlab function CAMFC2_Quad_New_02/Agent #2/Decenteralized Cooperaive Controller #2/Translational #2/Adaptive Law g_T #2 ==
  data: Agent_Num input; g_hat input; gama1 parameter; rho1 parameter; P input; P_struct parameter; Dg_hat output; e input; H parameter; N parameter; n parameter
function Dg_hat = fcn(Agent_Num,g_hat,gama1,rho1,P,P_struct,e,H,N,n)

P_struct(1).data = P.p1;
P_struct(2).data = P.p2;
P_struct(3).data = P.p3;
P_struct(4).data = P.p4;

Sum = zeros(n,1);
for i=1:N  
    Sum = Sum + (H(i,Agent_Num) * P_struct(i).data * e((i-1)*n+1:(i*n),1)); %Adaptive law
end
    
Dg_hat = -gama1*Sum - (rho1*gama1*g_hat);

end

== matlab function CAMFC2_Quad_New_02/Agent #2/Decenteralized Cooperaive Controller #2/Translational #2/DRE_T ==
  data: P input; A_hat input; B parameter; R parameter; DP output; Q parameter
function DP = fcn(P,A_hat,B,R,Q)

DP = 2*A_hat*P + 2*P*A_hat' - P*B*R*B'*P + 2*Q;

end

== matlab function CAMFC2_Quad_New_02/Agent #2/Decenteralized Cooperaive Controller #2/Translational #2/Differentiator1/Sliding differentiator ==
  data: u output; u1 input; e input; k1 parameter; alpha parameter
function u = fcn(u1,e,k1,alpha)

b=k1;

ABS = abs(e);
SGN = e ./ (ABS + alpha);
u = u1 - b*((ABS.^0.5).*SGN); 

end

== matlab function CAMFC2_Quad_New_02/Agent #2/Decenteralized Cooperaive Controller #2/Translational #2/Differentiator1/Sliding differentiator1 ==
  data: Du1 output; e input; k2 parameter; alpha parameter
function Du1 = fcn(e,k2,alpha)

a=k2;

ABS = abs(e);
SGN = e ./ (ABS + alpha);
Du1 = - a*SGN;

end

== matlab function CAMFC2_Quad_New_02/Agent #2/Decenteralized Cooperaive Controller #2/Translational #2/Main Controller_T #2 ==
  data: n parameter; n0 parameter; U output; R parameter; Q parameter; P_i input; e_i input; K parameter; Zeta_i input; BN parameter; A_hat_i input; u0 input; z0 input; DT_i input; T_i input; H parameter; q_i input; Agent_Num input; B_pseudo_inverse parameter; ui input; x0_hat_inp input; g_hat_i input; D_ui1 input
function U = fcn(n,n0,R,Q,P_i,e_i,K,Zeta_i,BN,A_hat_i,u0,z0,DT_i,T_i,H,q_i,Agent_Num,B_pseudo_inverse,ui,x0_hat_inp, g_hat_i, D_ui1)

D_eta_0 = [DT_i(1,:)';zeros(n0,1)];

%% 
z0_i = [z0;ui(1:n0)];
x0_hat_i = [x0_hat_inp;ui(1:n0)];
u0_i = [u0;D_ui1];

%%

S_H = sum(H(Agent_Num,:)) - H(Agent_Num,Agent_Num);
U4 = - S_H * ([q_i;u0_i(n0+1:n)] - [DT_i(1,:)';zeros(n0,1)] - (A_hat_i * (x0_hat_i - [T_i(1,:)';zeros(n0,1)])));
U1 = 1/2 * R * P_i * e_i; %Consensus Error
U5 = ( A_hat_i * ( H(Agent_Num,Agent_Num)*(2*x0_hat_i - 2*[T_i(1,:)';zeros(n0,1)] + [T_i(Agent_Num+1,:)';zeros(n0,1)]) ) ) - e_i;
U5(1:n0) = U5(1:n0) + ( BN(Agent_Num,Agent_Num) * z0_i(1:n0) );
U5(n0+1:n) = U5(n0+1:n) + ( 1 * z0_i(n0+1:n) );
U2 = - g_hat_i; %nonlinear compensation 
U3 = + [DT_i(Agent_Num+1,:)';zeros(n0,1)]; %Derivative of Formation parameters  
U6 = zeros(n,1);
U6(1:n0) = - BN(Agent_Num,Agent_Num)*( D_eta_0(1:n0) - u0_i(1:n0) ); %Connection to the leader
U6(n0+1:n) = - 1 * ( D_eta_0(n0+1:n) - u0_i(n0+1:n) );
U7 = K * Zeta_i; %Consensus time-integral
U8 = (2*Q - 3/4*R*P_i)*e_i;

U_input = U1 + U2 + U3 + U4 + U5 + U6 + U7 + U8;

U = B_pseudo_inverse * U_input / H(Agent_Num,Agent_Num);

end

== matlab function CAMFC2_Quad_New_02/Agent #2/Decenteralized Cooperaive Controller #2/Translational #2/Module to compute Consensus Error_T #2 ==
  data: T_i input; x input; x0 input; ep output; AN parameter; BN parameter; N parameter; n parameter; n0 parameter; Agent_Num input; ui input
function ep = fcn(T_i,x,x0,AN,BN,N,n,n0,Agent_Num,ui)

Diff_Star_to0 = (T_i((Agent_Num+1),:))';
Diff_Star_to_Other = (eye(n0) * Diff_Star_to0 * ones(1,N))' - T_i(2:N+1,:);
Diff_Star_to_Other = Diff_Star_to_Other';

xp = zeros(n,N);
for i=1:N
    xp(1:n,i) = [x((i-1)*(2*n)+1:(i-1)*(2*n)+n0);x((i-1)*(2*n)+(2*n0)+1:(i-1)*(2*n)+(2*n0)+n0)];
end

%%
xp_own = zeros(n,1);
xp_own(1:n,1) = xp(1:n,Agent_Num);

xp0 = [x0;ui(1:n0)];

xp_other = zeros(n,N);
ep = zeros(n,1);
ep(1:n0,1) = ep(1:n0,1) + ( BN(Agent_Num,Agent_Num)*(-(xp_own(1:n0)-xp0(1:n0))+Diff_Star_to0) );
ep(n0+1:n,1) = ep(n0+1:n,1) + ( 1*(-(xp_own(n0+1:n)-xp0(n0+1:n))) );

for i=1:N        
    xp_other(1:n,i) = xp(1:n,i);
    ep(1:n0,1) = ep(1:n0,1) + AN(Agent_Num,i)*(-(xp_own(1:n0)-xp_other(1:n0,i))+Diff_Star_to_Other(:,i));
    ep(n0+1:n,1) = ep(n0+1:n,1) + AN(Agent_Num,i)*(-(xp_own(n0+1:n)-xp_other(n0+1:n,i)));
end

end

== matlab function CAMFC2_Quad_New_02/Agent #4/Decenteralized Cooperaive Controller #4/Translational #4/Module to compute Consensus Error_T #4 ==
  data: T_i input; x input; x0 input; ep output; AN parameter; BN parameter; N parameter; n parameter; n0 parameter; Agent_Num input; ui input
function ep = fcn(T_i,x,x0,AN,BN,N,n,n0,Agent_Num,ui)

Diff_Star_to0 = (T_i((Agent_Num+1),:))';
Diff_Star_to_Other = (eye(n0) * Diff_Star_to0 * ones(1,N))' - T_i(2:N+1,:);
Diff_Star_to_Other = Diff_Star_to_Other';

xp = zeros(n,N);
for i=1:N
    xp(1:n,i) = [x((i-1)*(2*n)+1:(i-1)*(2*n)+n0);x((i-1)*(2*n)+(2*n0)+1:(i-1)*(2*n)+(2*n0)+n0)];
end

%%
xp_own = zeros(n,1);
xp_own(1:n,1) = xp(1:n,Agent_Num);

xp0 = [x0;ui(1:n0)];

xp_other = zeros(n,N);
ep = zeros(n,1);
ep(1:n0,1) = ep(1:n0,1) + ( BN(Agent_Num,Agent_Num)*(-(xp_own(1:n0)-xp0(1:n0))+Diff_Star_to0) );
ep(n0+1:n,1) = ep(n0+1:n,1) + ( 1*(-(xp_own(n0+1:n)-xp0(n0+1:n))) );

for i=1:N        
    xp_other(1:n,i) = xp(1:n,i);
    ep(1:n0,1) = ep(1:n0,1) + AN(Agent_Num,i)*(-(xp_own(1:n0)-xp_other(1:n0,i))+Diff_Star_to_Other(:,i));
    ep(n0+1:n,1) = ep(n0+1:n,1) + AN(Agent_Num,i)*(-(xp_own(n0+1:n)-xp_other(n0+1:n,i)));
end

end
